simulink model "lab2_3pi"  (R2020b)
settings: Solver=VariableStepAuto  StartTime=0.0  StopTime=10  RelTol=1e-3
settings Model: Creator=Dexp  LastModifiedBy=takem

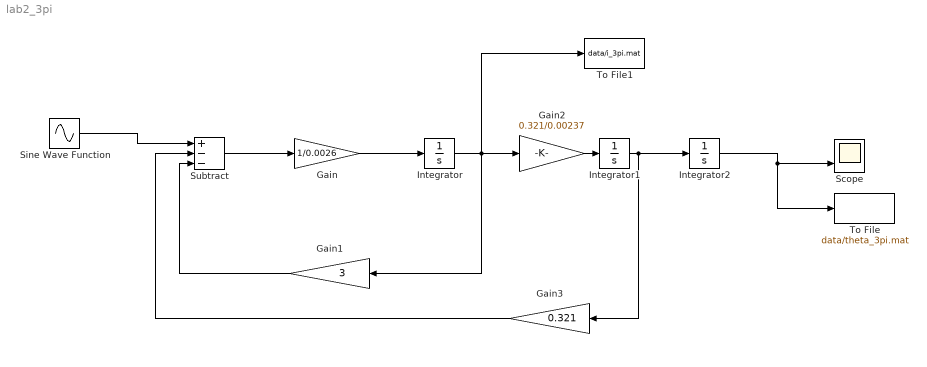
== system lab2_3pi ==
  Gain : Gain  Gain=1/0.0026
  Gain1 : Gain  Gain=3
  Gain2 : Gain  Gain=0.321/0.00237
  Gain3 : Gain  Gain=0.321
  Integrator : Integrator
  Integrator1 : Integrator
  Integrator2 : Integrator
  Scope : Scope  NumInputPorts=2
  Sine Wave Function : Sin  Amplitude=4.2  Frequency=3 * pi  SampleTime=0.01
  Subtract : Sum  Inputs=+--
  To File : ToFile  Filename=data/theta_3pi.mat  MatrixName=theta_3pi
  To File1 : ToFile  Filename=data/i_3pi.mat  MatrixName=i_3pi
  wires:
  Subtract/1 -> Gain/1
  Gain/1 -> Integrator/1
  Integrator/1 -> To File1/1, Gain2/1, Gain1/1
  Integrator1/1 -> Integrator2/1, Gain3/1
  Gain1/1 -> Subtract/3
  Gain2/1 -> Integrator1/1
  Gain3/1 -> Subtract/2
  Integrator2/1 -> Scope/2, To File/1
  Sine Wave Function/1 -> Subtract/1
